simulink model "odev3_iremelmas_kara"  (R2023b)
settings: Solver=ode23tb  StartTime=0.0  StopTime=0.104  MaxStep=1e-6  RelTol=1e-3
libraries: spsMeanLib x5, spsCurrentMeasurementLib x3, spsVoltageMeasurementLib x3, spsSeriesRLCBranchLib x2, spsDiodeLib x1, spsDCVoltageSourceLib x1, spsLinearTransformerLib x1, spsIGBTLib x1, spsRMSLib x1, spspowerguiLib x1
settings Model: Creator=ireme  LastModifiedBy=ireme

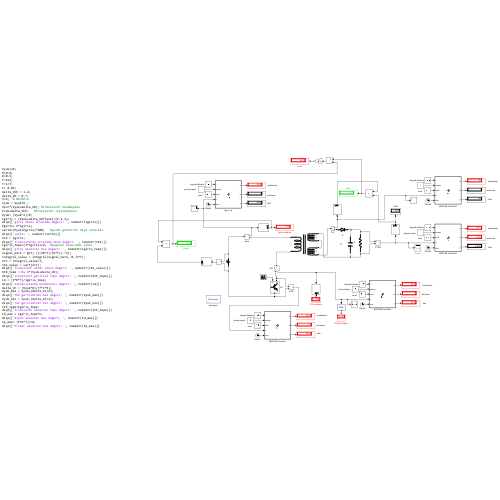
[thumbnail: Simulink's stored preview of the top-level diagram]
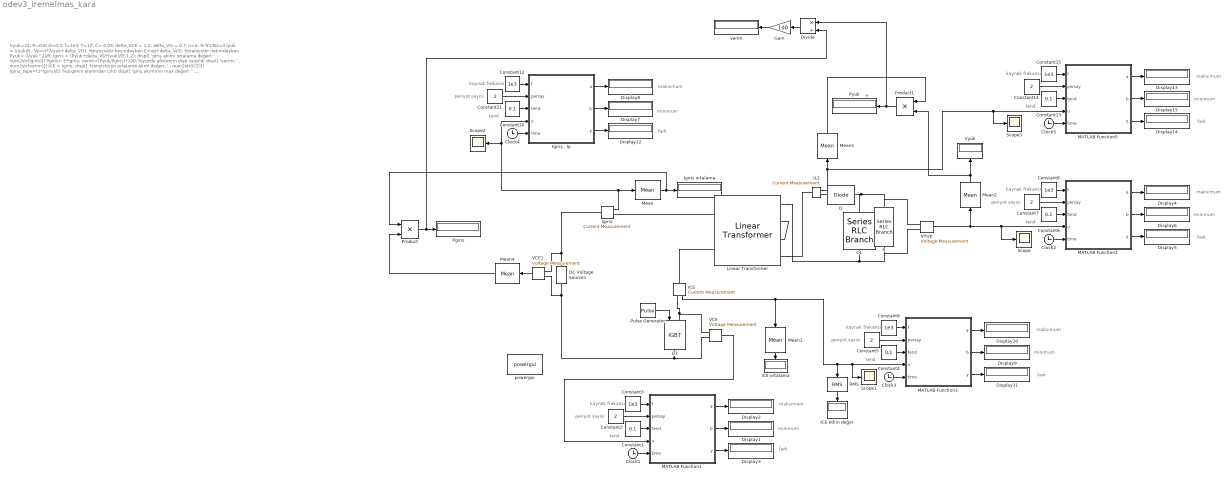
== system odev3_iremelmas_kara ==
  note: Vyuk=24;
      | R=0.8;
      | D=0.5;
      | f=1e3;
      | T=1/f;
      | C= 0.03;
      | delta_VCE = 1.2;
      | delta_VD = 0.7;
      | n=4; % N1/N2=4
      | Iyuk = Vyuk/R ;
      | Vp=n*(Vyuk+delta_VD); %tranzistör kesmdeyken
      | E=Vp+delta_VCE; %tranzistör iletimdeyken
      | Pyuk= (Vyuk^2)/R;
      | Igiris = (Pyuk+delta_VD*Iyuk)/(E-1.2);
      | disp([ 'giriş akımı ortalama değeri: ' , num2str(Igiris)])
      | Pgiris= E*Igiris;
      | verim=(Pyuk/Pgiris)*100; %yuzde göstersin diye carpıldı
      | disp([ 'verim: ' , num2str(verim)])
      | ICE = Igiris;
      | disp([ 'transistörün ortalama akım değeri: ' , num2str(ICE)])
      | Igiris_tepe=(2*Igiris)/D; %ücgenin alanından çıktı
      | disp([ 'giriş akımının max değeri: ' , num2str(Igiris_tepe)])
      | signal_kare = @(t) (((30*t)/(D*T)).^2);
      | integral_value = integral(signal_kare, 0, D*T);
      | ort = integral_value/T;
      | rms_value = sqrt(ort);
      | disp([ 'transistör akımı etkin değeri: ' , num2str(rms_value)])
      | VCE_tepe = E+ n*(Vyuk+delta_VD);
      | disp([ 'transistör gerilimi tepe değeri: ' , num2str(VCE_tepe)])
      | Lm = (E*D*T)/Igiris_tepe;
      | disp([ 'mıknatıslanma endüktansı değeri: ' , num2str(Lm)])
      | delta_VC = (Vyuk*D)/(f*C*R);
      | Vyuk_max = Vyuk+(delta_VC/2);
      | disp([ 'Yük geriliminin max değeri: ' , num2str(Vyuk_max)])
      | Vyuk_min = Vyuk-(delta_VC/2);
      | disp([ 'Yük geriliminin min değeri: ' , num2str(Vyuk_min)])
      | ICE_tepe=Igiris_tepe;
      | disp([ 'transistör akımının tepe değeri: ' , num2str(ICE_tepe)])
      | Id_max = Igiris_tepe*n;
      | disp([ 'diyot akımının max değeri: ' , num2str(Id_max)])
      | Ip_max= (E*D*T)/Lm;
      | disp([ 'Primer akımının max değeri: ' , num2str(Ip_max)])
  note: a
  note: maksimum
  note: kaynak frekansi
  note: periyot sayisi
  note: minimum
  note: fark
  note: tend
  note: minimum
  note: fark
  note: tend
  note: periyot sayisi
  note: kaynak frekansi
  note: maksimum
  note: periyot sayisi
  note: maksimum
  note: minimum
  note: fark
  note: kaynak frekansi
  note: tend
  note: minimum
  note: kaynak frekansi
  note: tend
  note: maksimum
  note: fark
  note: periyot sayisi
  note: fark
  note: tend
  note: minimum
  note: kaynak frekansi
  note: maksimum
  C1 : spsSeriesRLCBranchLib/Series RLC Branch  LConnTagsString=__new0  RConnTagsString=__new0  BranchType=C  Resistance=1  Inductance=180e-6  SetiL0=off  InitialCurrent=0  Capacitance=0.03  Setx0=off  InitialVoltage=0  Measurements=None
  Clock{1..5} (5 alike) : Clock
      settings: Decimation=100
  Constant{1,4,6,10,13} (5 alike) : Constant  Value=0.1  SampleTime=0
  Constant{2,5,7,11,14} (5 alike) : Constant  Value=2  SampleTime=0
  Constant{3,8..9,12,15} (5 alike) : Constant  Value=1e3  SampleTime=0
  D : spsDiodeLib/Diode  Ron=1e-10  Lon=0  Vf=0.7  IC=0  UseSnubber=off  Rs=5000  Cs=250e-6  Measurements=off
  DC Voltage Source1 : spsDCVoltageSourceLib/DC Voltage Source  Amplitude=100  Measurements=Voltage
  Display{1..15} (15 alike) : Display
  Divide : Product  Inputs=*/
  Gain : Gain  Gain=100
  ICE : spsCurrentMeasurementLib/Current Measurement  PhasorSimulation=off  OutputType=Complex  PSBequivalent=0
  ICE etkin değer : Display
  ICE ortalama : Display
  IL2 : spsCurrentMeasurementLib/Current Measurement  PhasorSimulation=off  OutputType=Complex  PSBequivalent=0
  Igiris : spsCurrentMeasurementLib/Current Measurement  PhasorSimulation=off  OutputType=Complex  PSBequivalent=0
  Igiris ortalama : Display
  "Igiriş , Ip" : MATLAB Function  TreatAsAtomicUnit=on
  Linear Transformer : spsLinearTransformerLib/Linear Transformer  UNITS=SI  NominalPower=[1000 50]  winding1=[100 0 0]  winding2=[12 0 0]  ThreeWindings=on  winding3=[12 0 0]  RmLm=[1e6 1.67e-3]  Measurements=None  DataType=on
  MATLAB Function1 : MATLAB Function  TreatAsAtomicUnit=on
  MATLAB Function2 : MATLAB Function  TreatAsAtomicUnit=on
  MATLAB Function3 : MATLAB Function  TreatAsAtomicUnit=on
  MATLAB Function5 : MATLAB Function  TreatAsAtomicUnit=on
  Mean{,1..2,4..5} (5 alike) : spsMeanLib/Mean  Freq=1e3  Vinit=0  Ts=0
  Pgiris : Display
  Product : Product
  Product1 : Product
  Pulse Generator : DiscretePulseGenerator  PulseType=Time based  Period=1e-3  PulseWidth=50
  Pyuk : Display
  Q1 : spsIGBTLib/IGBT  Ron=1e-8  Lon=0  Vf=1.2  Tf=1e-6  Tt=2e-6  IC=0  Rs=1e5  Cs=inf  Measurements=off
  R : spsSeriesRLCBranchLib/Series RLC Branch  LConnTagsString=__new0  RConnTagsString=__new0  BranchType=R  Resistance=0.8  Inductance=180e-6  SetiL0=off  InitialCurrent=0  Capacitance=1e-6  Setx0=off  InitialVoltage=0  Measurements=None
  RMS : spsRMSLib/RMS  TrueRMS=on  Freq=60  RMSInit=120  Ts=0
  Scope{,1..3} (4 alike) : Scope
  VCE : spsVoltageMeasurementLib/Voltage Measurement  PhasorSimulation=off  OutputType=Complex  PSBequivalent=0
  VCE1 : spsVoltageMeasurementLib/Voltage Measurement  PhasorSimulation=off  OutputType=Complex  PSBequivalent=0
  VYUK : spsVoltageMeasurementLib/Voltage Measurement  PhasorSimulation=off  OutputType=Complex  PSBequivalent=0
  Vyük : Display
  powergui : spspowerguiLib/powergui  Priority=1  SimulationMode=Continuous  SampleTime=50e-8  frequency=60  Iterations=50  frequencyindice=0  Pbase=100e6  ErrMax=1e-4  UnitsV=kV  UnitsW=MW  buscounter=0  FunctionMessages=off  echomessages=off  EnableUseOfTLC=off  CurrentSourceSwitches=off  DisableSnubberDevices=on  DisableRonSwitches=off  DisableVfSwitches=off  DisplayEquations=off  AutomaticDiscreteSolvers=off  SolverType=Tustin/Backward Euler (TBE)  Interpol=off  ExternalGateDelay=off  methode=off  Ts=100  x0status=zero  SPID=off  SwTol=0  HookPort=off  NonlinearTolerance=0  nMaxIteration=15  ContinueOnMaxIteration=off  RestoreLinks=warning  ResistiveCurrentMeasurement=off  Frange=[0:2:500]  Ylog=off  Xlog=on  ShowGrid=off  save=off  variable=ZData  structure=0  ZoomFFT=off  StartTime=0.0  cycles=1  DisplayStyle=1  fundamental=60  FreqAxis=off  MaxFrequency=1000  frequencyindicesteady=1  RmsSteady=1  display=off
  verim : Display
  wires:
  Pulse Generator/1 -> Q1/1
  Igiris/1 -> Mean/1, Scope2/1, "Igiriş , Ip"/4(u)
  Clock1/1 -> MATLAB Function1/5(time)
  MATLAB Function1/2(b) -> Display1/1
  Constant1/1 -> MATLAB Function1/3(tend)
  Constant2/1 -> MATLAB Function1/2(persay)
  Constant3/1 -> MATLAB Function1/1(f)
  MATLAB Function1/1(a) -> Display2/1
  MATLAB Function1/3(y) -> Display3/1
  VCE/1 -> MATLAB Function1/4(u)
  Constant9/1 -> MATLAB Function3/1(f)
  Clock3/1 -> MATLAB Function3/5(time)
  Constant5/1 -> MATLAB Function3/2(persay)
  MATLAB Function3/2(b) -> Display9/1
  MATLAB Function3/1(a) -> Display10/1
  Constant4/1 -> MATLAB Function3/3(tend)
  MATLAB Function3/3(y) -> Display11/1
  Mean1/1 -> ICE ortalama/1
  ICE/1 -> RMS/1, Scope1/1, MATLAB Function3/4(u), Mean1/1
  Mean2/1 -> Product1/2, Vyük/1
  Product1/1 -> Divide/1, Pyuk/1
  Divide/1 -> Gain/1
  Gain/1 -> verim/1
  MATLAB Function2/3(y) -> Display5/1
  Clock2/1 -> MATLAB Function2/5(time)
  Constant7/1 -> MATLAB Function2/2(persay)
  MATLAB Function2/1(a) -> Display4/1
  Constant8/1 -> MATLAB Function2/1(f)
  MATLAB Function2/2(b) -> Display6/1
  Constant6/1 -> MATLAB Function2/3(tend)
  Constant12/1 -> "Igiriş , Ip"/1(f)
  "Igiriş , Ip"/3(y) -> Display12/1
  "Igiriş , Ip"/1(a) -> Display8/1
  Constant10/1 -> "Igiriş , Ip"/3(tend)
  "Igiriş , Ip"/2(b) -> Display7/1
  Constant11/1 -> "Igiriş , Ip"/2(persay)
  Clock4/1 -> "Igiriş , Ip"/5(time)
  VCE1/1 -> Mean4/1
  Constant15/1 -> MATLAB Function5/1(f)
  MATLAB Function5/1(a) -> Display13/1
  Clock5/1 -> MATLAB Function5/5(time)
  Constant14/1 -> MATLAB Function5/2(persay)
  MATLAB Function5/3(y) -> Display14/1
  MATLAB Function5/2(b) -> Display15/1
  Constant13/1 -> MATLAB Function5/3(tend)
  RMS/1 -> ICE etkin değer/1
  Product/1 -> Divide/2, Pgiris/1
  Mean4/1 -> Product/2
  Mean/1 -> Igiris ortalama/1, Product/1
  VYUK/1 -> Scope/1, MATLAB Function2/4(u), Mean2/1
  IL2/1 -> Mean5/1, Scope3/1, MATLAB Function5/4(u)
  Mean5/1 -> Product1/1
  connections:
  D/RConn1 -- VYUK/LConn1 -- R/LConn1 -- C1/LConn1
  Linear Transformer/RConn1 -- R/RConn1 -- VYUK/LConn2 -- C1/RConn1
  Q1/RConn1 -- VCE/LConn2 -- VCE1/LConn2 -- DC Voltage Source1/LConn1
  ICE/LConn1 -- Linear Transformer/LConn2
  Linear Transformer/RConn2 -- Linear Transformer/RConn3
  Igiris/RConn1 -- Linear Transformer/LConn1
  DC Voltage Source1/RConn1 -- VCE1/LConn1 -- Igiris/LConn1
  D/LConn1 -- IL2/RConn1
  Linear Transformer/RConn4 -- IL2/LConn1
  ICE/RConn1 -- VCE/LConn1 -- Q1/LConn1

== matlab function odev3_iremelmas_kara/MATLAB Function1 ==
  settings: updateMethod=DISCRETE
  data: a output; b output; f input; persay input; tend input; u input; y output; time input
function [a,b,y] = fcn(f,persay,tend,u,time)
% persistent değişken; değişken değerini kalıcı olarak tutar ve direk atama
% yapılmadıkça değişmez. Normal değişkenler fonksiyonun her yenilenme 
% durumunda sıfırlanırken, persistent değişkeni, kalıcı olması sebebiyle,
% bir önceki değeri tutabilme yeteneğine sahiptir. 
% Bu da bize bir önceki değer ile güncel değerinizi karşılaştırma olanağı
% sunar.
a=1/0;b=0;
persistent enbuyuk;
persistent enkucuk;
persistent fark;
% Eğer persistent değişkenini en başta persistent enbuyuk = 0; olarak 
% tanımlarsak, sürekli 0 olarak kalacaktır. Aynı zamanda eğer bir ilk değer 
% vermezseniz "null" değerini taşıyacağından, if yapılarında hata
% verecektir. Bu hatadan kaçınmak için, isempty komutu ile persistent
% değişkenlerinin "null" olup olmadığını kontrol edilir ve ilk değer ataması
% yapılır. Bu değişkenler sadece  fonksiyon ilk kez çalıştığında
% null olacağı için(daha sonra sürekli gelen değeri tuttuğu yukarıda söylenmişti)
% başlangıçta, bir kereye mahsus olarak,  aşağıdaki if yapısı doğrulanacak 
% ve değişkenlere ilk değerler atanacaktır.
%
if (isempty(enkucuk) || isempty(enbuyuk))  
enkucuk = 1/0;   
enbuyuk = 0;
end
if (time>tend-(persay+1)*1/f) && (time<=tend) % Periyot ~= 0.01 // Son iki periyodu hesaplar.
    if u >= enbuyuk
        enbuyuk = u;
     end
    if u < enkucuk   
        enkucuk = u;
    end
end
fark = enbuyuk - enkucuk;
a=enbuyuk;
b=enkucuk;
y=fark;
end

== matlab function odev3_iremelmas_kara/MATLAB Function3 ==
  settings: updateMethod=DISCRETE
  data: a output; b output; f input; persay input; tend input; u input; y output; time input
function [a,b,y] = fcn(f,persay,tend,u,time)
% persistent değişken; değişken değerini kalıcı olarak tutar ve direk atama
% yapılmadıkça değişmez. Normal değişkenler fonksiyonun her yenilenme 
% durumunda sıfırlanırken, persistent değişkeni, kalıcı olması sebebiyle,
% bir önceki değeri tutabilme yeteneğine sahiptir. 
% Bu da bize bir önceki değer ile güncel değerinizi karşılaştırma olanağı
% sunar.
a=1/0;b=0;
persistent enbuyuk;
persistent enkucuk;
persistent fark;
% Eğer persistent değişkenini en başta persistent enbuyuk = 0; olarak 
% tanımlarsak, sürekli 0 olarak kalacaktır. Aynı zamanda eğer bir ilk değer 
% vermezseniz "null" değerini taşıyacağından, if yapılarında hata
% verecektir. Bu hatadan kaçınmak için, isempty komutu ile persistent
% değişkenlerinin "null" olup olmadığını kontrol edilir ve ilk değer ataması
% yapılır. Bu değişkenler sadece  fonksiyon ilk kez çalıştığında
% null olacağı için(daha sonra sürekli gelen değeri tuttuğu yukarıda söylenmişti)
% başlangıçta, bir kereye mahsus olarak,  aşağıdaki if yapısı doğrulanacak 
% ve değişkenlere ilk değerler atanacaktır.
%
if (isempty(enkucuk) || isempty(enbuyuk))  
enkucuk = 1/0;   
enbuyuk = 0;
end
if (time>tend-(persay+1)*1/f) && (time<=tend) % Periyot ~= 0.01 // Son iki periyodu hesaplar.
    if u >= enbuyuk
        enbuyuk = u;
     end
    if u < enkucuk   
        enkucuk = u;
    end
end
fark = enbuyuk - enkucuk;
a=enbuyuk;
b=enkucuk;
y=fark;
end

== matlab function odev3_iremelmas_kara/MATLAB Function2 ==
  settings: updateMethod=DISCRETE
  data: a output; b output; f input; persay input; tend input; u input; y output; time input
function [a,b,y] = fcn(f,persay,tend,u,time)
% persistent değişken; değişken değerini kalıcı olarak tutar ve direk atama
% yapılmadıkça değişmez. Normal değişkenler fonksiyonun her yenilenme 
% durumunda sıfırlanırken, persistent değişkeni, kalıcı olması sebebiyle,
% bir önceki değeri tutabilme yeteneğine sahiptir. 
% Bu da bize bir önceki değer ile güncel değerinizi karşılaştırma olanağı
% sunar.
a=1/0;b=0;
persistent enbuyuk;
persistent enkucuk;
persistent fark;
% Eğer persistent değişkenini en başta persistent enbuyuk = 0; olarak 
% tanımlarsak, sürekli 0 olarak kalacaktır. Aynı zamanda eğer bir ilk değer 
% vermezseniz "null" değerini taşıyacağından, if yapılarında hata
% verecektir. Bu hatadan kaçınmak için, isempty komutu ile persistent
% değişkenlerinin "null" olup olmadığını kontrol edilir ve ilk değer ataması
% yapılır. Bu değişkenler sadece  fonksiyon ilk kez çalıştığında
% null olacağı için(daha sonra sürekli gelen değeri tuttuğu yukarıda söylenmişti)
% başlangıçta, bir kereye mahsus olarak,  aşağıdaki if yapısı doğrulanacak 
% ve değişkenlere ilk değerler atanacaktır.
%
if (isempty(enkucuk) || isempty(enbuyuk))  
enkucuk = 1/0;   
enbuyuk = 0;
end
if (time>tend-(persay+1)*1/f) && (time<=tend) % Periyot ~= 0.01 // Son iki periyodu hesaplar.
    if u >= enbuyuk
        enbuyuk = u;
     end
    if u < enkucuk   
        enkucuk = u;
    end
end
fark = enbuyuk - enkucuk;
a=enbuyuk;
b=enkucuk;
y=fark;
end

== matlab function odev3_iremelmas_kara/Igiriş , Ip ==
  settings: updateMethod=DISCRETE
  data: a output; b output; f input; persay input; tend input; u input; y output; time input
function [a,b,y] = fcn(f,persay,tend,u,time)
% persistent değişken; değişken değerini kalıcı olarak tutar ve direk atama
% yapılmadıkça değişmez. Normal değişkenler fonksiyonun her yenilenme 
% durumunda sıfırlanırken, persistent değişkeni, kalıcı olması sebebiyle,
% bir önceki değeri tutabilme yeteneğine sahiptir. 
% Bu da bize bir önceki değer ile güncel değerinizi karşılaştırma olanağı
% sunar.
a=1/0;b=0;
persistent enbuyuk;
persistent enkucuk;
persistent fark;
% Eğer persistent değişkenini en başta persistent enbuyuk = 0; olarak 
% tanımlarsak, sürekli 0 olarak kalacaktır. Aynı zamanda eğer bir ilk değer 
% vermezseniz "null" değerini taşıyacağından, if yapılarında hata
% verecektir. Bu hatadan kaçınmak için, isempty komutu ile persistent
% değişkenlerinin "null" olup olmadığını kontrol edilir ve ilk değer ataması
% yapılır. Bu değişkenler sadece  fonksiyon ilk kez çalıştığında
% null olacağı için(daha sonra sürekli gelen değeri tuttuğu yukarıda söylenmişti)
% başlangıçta, bir kereye mahsus olarak,  aşağıdaki if yapısı doğrulanacak 
% ve değişkenlere ilk değerler atanacaktır.
%
if (isempty(enkucuk) || isempty(enbuyuk))  
enkucuk = 1/0;   
enbuyuk = 0;
end
if (time>tend-(persay+1)*1/f) && (time<=tend) % Periyot ~= 0.01 // Son iki periyodu hesaplar.
    if u >= enbuyuk
        enbuyuk = u;
     end
    if u < enkucuk   
        enkucuk = u;
    end
end
fark = enbuyuk - enkucuk;
a=enbuyuk;
b=enkucuk;
y=fark;
end

== matlab function odev3_iremelmas_kara/MATLAB Function5 ==
  settings: updateMethod=DISCRETE
  data: a output; b output; f input; persay input; tend input; u input; y output; time input
function [a,b,y] = fcn(f,persay,tend,u,time)
% persistent değişken; değişken değerini kalıcı olarak tutar ve direk atama
% yapılmadıkça değişmez. Normal değişkenler fonksiyonun her yenilenme 
% durumunda sıfırlanırken, persistent değişkeni, kalıcı olması sebebiyle,
% bir önceki değeri tutabilme yeteneğine sahiptir. 
% Bu da bize bir önceki değer ile güncel değerinizi karşılaştırma olanağı
% sunar.
a=1/0;b=0;
persistent enbuyuk;
persistent enkucuk;
persistent fark;
% Eğer persistent değişkenini en başta persistent enbuyuk = 0; olarak 
% tanımlarsak, sürekli 0 olarak kalacaktır. Aynı zamanda eğer bir ilk değer 
% vermezseniz "null" değerini taşıyacağından, if yapılarında hata
% verecektir. Bu hatadan kaçınmak için, isempty komutu ile persistent
% değişkenlerinin "null" olup olmadığını kontrol edilir ve ilk değer ataması
% yapılır. Bu değişkenler sadece  fonksiyon ilk kez çalıştığında
% null olacağı için(daha sonra sürekli gelen değeri tuttuğu yukarıda söylenmişti)
% başlangıçta, bir kereye mahsus olarak,  aşağıdaki if yapısı doğrulanacak 
% ve değişkenlere ilk değerler atanacaktır.
%
if (isempty(enkucuk) || isempty(enbuyuk))  
enkucuk = 1/0;   
enbuyuk = 0;
end
if (time>tend-(persay+1)*1/f) && (time<=tend) % Periyot ~= 0.01 // Son iki periyodu hesaplar.
    if u >= enbuyuk
        enbuyuk = u;
     end
    if u < enkucuk   
        enkucuk = u;
    end
end
fark = enbuyuk - enkucuk;
a=enbuyuk;
b=enkucuk;
y=fark;
end
